simulink library "WBCLibrary"  (R2014b)
settings: Solver=ode45  StartTime=0.0  StopTime=10.0  RelTol=1e-3
undefined symbols (not defined in the file or in its folder): LinkName, localName, ROBOT_DOF, robotName, Ts
undefined symbols (not defined in the file): Tt
libraries: WBCLibrary x10, simulink x1
(part 2 of 2)

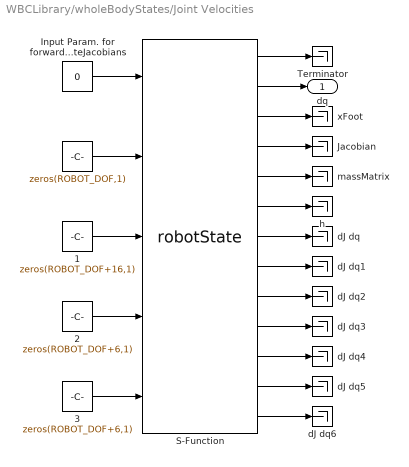
== system WBCLibrary/wholeBodyStates/Joint Velocities ==
  " " : Constant  Value=zeros(ROBOT_DOF,1)  OutDataTypeStr=double  SampleTime=Ts
  " 1" : Constant  Value=zeros(ROBOT_DOF+16,1)  OutDataTypeStr=double  SampleTime=Ts
  " 2" : Constant  Value=zeros(ROBOT_DOF+6,1)  OutDataTypeStr=double  SampleTime=Ts
  " 3" : Constant  Value=zeros(ROBOT_DOF+6,1)  OutDataTypeStr=double  SampleTime=Ts
  "Input Param. for forwardKinematics and computeJacobians " : Constant  Value=0  OutDataTypeStr=int8  SampleTime=Ts
  Jacobian : Terminator
  S-Function : S-Function  FunctionName=robotState  Parameters=val,robotname,localname,linkname  EnableBusSupport=off  mask{val=1, robotname=robotName, localname=localName, linkname='na'}
      mask prompts: val "Value"; robotname "Robot Name (icub - icubSim)"; localname "Module Name"; linkname "Link Name"
  Terminator : Terminator
  dJ dq{,1..6} (7 alike) : Terminator
  h : Terminator
  massMatrix : Terminator
  xFoot : Terminator
  dq : Outport
  wires:
  " "/1 -> S-Function/2
  S-Function/2 -> dq/1
  S-Function/1 -> Terminator/1
  S-Function/3 -> xFoot/1
  "Input Param. for forwardKinematics and computeJacobians "/1 -> S-Function/1
  S-Function/4 -> Jacobian/1
  S-Function/5 -> massMatrix/1
  S-Function/6 -> h/1
  S-Function/7 -> dJ dq/1
  S-Function/8 -> dJ dq1/1
  S-Function/9 -> dJ dq2/1
  S-Function/10 -> dJ dq3/1
  " 1"/1 -> S-Function/3
  " 2"/1 -> S-Function/4
  " 3"/1 -> S-Function/5
  S-Function/11 -> dJ dq4/1
  S-Function/12 -> dJ dq5/1
  S-Function/13 -> dJ dq6/1

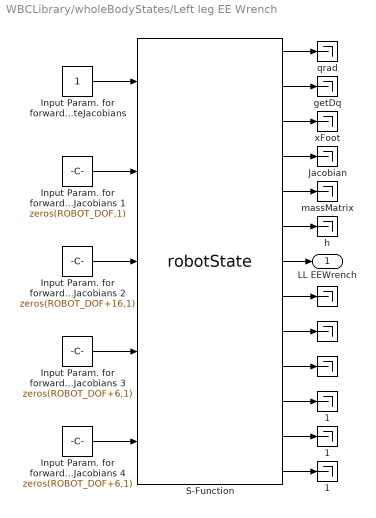
== system WBCLibrary/wholeBodyStates/Left leg EE Wrench ==
  " " : Terminator
  "  " : Terminator
  "   " : Terminator
  "   1" : Terminator
  "  1" : Terminator
  " 1" : Terminator
  "Input Param. for forwardKinematics and computeJacobians " : Constant  OutDataTypeStr=int8  SampleTime=Ts
  Input Param. for forwardKinematics and computeJacobians 1 : Constant  Value=zeros(ROBOT_DOF,1)  OutDataTypeStr=double  SampleTime=Ts
  Input Param. for forwardKinematics and computeJacobians 2 : Constant  Value=zeros(ROBOT_DOF+16,1)  OutDataTypeStr=double  SampleTime=Ts
  Input Param. for forwardKinematics and computeJacobians 3 : Constant  Value=zeros(ROBOT_DOF+6,1)  OutDataTypeStr=double  SampleTime=Ts
  Input Param. for forwardKinematics and computeJacobians 4 : Constant  Value=zeros(ROBOT_DOF+6,1)  OutDataTypeStr=double  SampleTime=Ts
  Jacobian : Terminator
  S-Function : S-Function  FunctionName=robotState  Parameters=val,robotname,localname,linkname  EnableBusSupport=off  mask{val=15, robotname=robotName, localname=localName, linkname='l_sole'}
      mask prompts: val "Value"; robotname "Robot Name (icub - icubSim)"; localname "Module Name"; linkname "Link Name"
  getDq : Terminator
  h : Terminator
  massMatrix : Terminator
  qrad : Terminator
  xFoot : Terminator
  LL EEWrench : Outport
  wires:
  Input Param. for forwardKinematics and computeJacobians 4/1 -> S-Function/5
  Input Param. for forwardKinematics and computeJacobians 3/1 -> S-Function/4
  Input Param. for forwardKinematics and computeJacobians 2/1 -> S-Function/3
  S-Function/10 -> "   "/1
  S-Function/9 -> "  "/1
  S-Function/8 -> " "/1
  S-Function/7 -> LL EEWrench/1
  S-Function/6 -> h/1
  S-Function/5 -> massMatrix/1
  S-Function/4 -> Jacobian/1
  "Input Param. for forwardKinematics and computeJacobians "/1 -> S-Function/1
  S-Function/3 -> xFoot/1
  S-Function/1 -> qrad/1
  S-Function/2 -> getDq/1
  Input Param. for forwardKinematics and computeJacobians 1/1 -> S-Function/2
  S-Function/11 -> " 1"/1
  S-Function/12 -> "  1"/1
  S-Function/13 -> "   1"/1

== system WBCLibrary/wholeBodyStates/Right leg EE Wrench ==
  " " : Constant  Value=zeros(ROBOT_DOF,1)  OutDataTypeStr=double  SampleTime=-1
  " 1" : Constant  Value=zeros(ROBOT_DOF+16,1)  OutDataTypeStr=double  SampleTime=-1
  " 2" : Constant  Value=zeros(ROBOT_DOF+6,1)  OutDataTypeStr=double  SampleTime=-1
  " 3" : Constant  Value=zeros(ROBOT_DOF+6,1)  OutDataTypeStr=double  SampleTime=-1
  "Input Param. for forwardKinematics and computeJacobians " : Constant  Value=0  OutDataTypeStr=int8
  Jacobian : Terminator
  S-Function : S-Function  FunctionName=robotState  Parameters=val,robotname,localname,linkname  EnableBusSupport=off  mask{val=15, robotname=robotName, localname=localName, linkname='r_sole'}
      mask prompts: val "Value"; robotname "Robot Name (icub - icubSim)"; localname "Module Name"; linkname "Link Name"
  Terminator : Terminator
  Terminator1 : Terminator
  dJ dq{1..6} (6 alike) : Terminator
  h : Terminator
  massMatrix : Terminator
  xFoot : Terminator
  RL EEWrench : Outport
  wires:
  " 3"/1 -> S-Function/5
  " 2"/1 -> S-Function/4
  " 1"/1 -> S-Function/3
  S-Function/10 -> dJ dq3/1
  S-Function/9 -> dJ dq2/1
  S-Function/8 -> dJ dq1/1
  S-Function/7 -> RL EEWrench/1
  S-Function/6 -> h/1
  S-Function/5 -> massMatrix/1
  S-Function/4 -> Jacobian/1
  "Input Param. for forwardKinematics and computeJacobians "/1 -> S-Function/1
  S-Function/3 -> xFoot/1
  S-Function/1 -> Terminator/1
  S-Function/2 -> Terminator1/1
  " "/1 -> S-Function/2
  S-Function/13 -> dJ dq6/1
  S-Function/12 -> dJ dq5/1
  S-Function/11 -> dJ dq4/1

== system WBCLibrary/wholeBodyStates/dq_b + dq_j ==
  Joint Velocities : WBCLibrary/wholeBodyStates/Joint Velocities  robotName=robotName  localName=localName
  Left Foot Jacobian : WBCLibrary/wholeBodyModel/Jacobians/Left Foot Jacobian  robotName=robotName  localName=localName
  Mux : Mux  Inputs=2
  Right Foot Jacobian : WBCLibrary/wholeBodyModel/Jacobians/Right Foot Jacobian  robotName=robotName  localName=localName
  baseVelocity : WBCLibrary/Utilities/baseVelocity
  dq : Outport
  wires:
  Mux/1 -> dq/1
  Joint Velocities/1 -> Mux/2, baseVelocity/3
  baseVelocity/1 -> Mux/1
  Right Foot Jacobian/1 -> baseVelocity/1
  Left Foot Jacobian/1 -> baseVelocity/2

== system WBCLibrary/wholeBodyStates/q_b + q_j ==
  Constant1 : Constant  Value=zeros(16,1)
  Joint Angles : WBCLibrary/wholeBodyStates/Joint Angles  robotName=robotName  localName=localName
  Mux : Mux  Inputs=2
  q : Outport
  wires:
  Constant1/1 -> Mux/1
  Joint Angles/1 -> Mux/2
  Mux/1 -> q/1

== system WBCLibrary/wholeBodyModel/Dynamics/Cent Momentum ==
  q : Inport
  dq : Inport  Port=2
  RightFoot : Constant  Value=0  OutDataTypeStr=int8  SampleTime=Ts
  S-Function : S-Function  FunctionName=robotState  Parameters=14,robotName,localName,'na'  EnableBusSupport=off
  Terminator{,1..11} (12 alike) : Terminator
  dummy : Constant  Value=zeros(ROBOT_DOF,1)  OutDataTypeStr=double  SampleTime=Ts
  dummy3 : Constant  Value=zeros(ROBOT_DOF+6,1)  OutDataTypeStr=double  SampleTime=Ts
  H : Outport
  wires:
  S-Function/13 -> H/1
  dummy3/1 -> S-Function/5
  dq/1 -> S-Function/4
  q/1 -> S-Function/3
  dummy/1 -> S-Function/2
  RightFoot/1 -> S-Function/1
  S-Function/12 -> Terminator11/1
  S-Function/11 -> Terminator10/1
  S-Function/10 -> Terminator9/1
  S-Function/9 -> Terminator8/1
  S-Function/8 -> Terminator7/1
  S-Function/7 -> Terminator6/1
  S-Function/6 -> Terminator5/1
  S-Function/5 -> Terminator4/1
  S-Function/4 -> Terminator3/1
  S-Function/3 -> Terminator2/1
  S-Function/2 -> Terminator1/1
  S-Function/1 -> Terminator/1

== system WBCLibrary/wholeBodyModel/Dynamics/Inverse Dynamics ==
  q : Inport
  dq : Inport  Port=2
  ddq : Inport  Port=3
  Constant : Constant  Value=zeros(ROBOT_DOF,1)  OutDataTypeStr=double  SampleTime=Ts
  Constant2 : Constant  Value=0  OutDataTypeStr=int8  SampleTime=Ts
  S-Function : S-Function  FunctionName=robotState  Parameters=12,robotName,localName,'na'  EnableBusSupport=off
  Terminator{,1..11} (12 alike) : Terminator
  genTau : Outport
  wires:
  S-Function/10 -> genTau/1
  S-Function/9 -> Terminator8/1
  Constant/1 -> S-Function/2
  Constant2/1 -> S-Function/1
  q/1 -> S-Function/3
  dq/1 -> S-Function/4
  ddq/1 -> S-Function/5
  S-Function/1 -> Terminator/1
  S-Function/2 -> Terminator1/1
  S-Function/3 -> Terminator2/1
  S-Function/4 -> Terminator3/1
  S-Function/5 -> Terminator4/1
  S-Function/6 -> Terminator5/1
  S-Function/7 -> Terminator6/1
  S-Function/8 -> Terminator7/1
  S-Function/11 -> Terminator9/1
  S-Function/12 -> Terminator10/1
  S-Function/13 -> Terminator11/1

== system WBCLibrary/wholeBodyModel/Dynamics/computeh ==
  q : Inport
  dq : Inport  Port=2
  " " : Terminator
  "  " : Terminator
  "  1" : Terminator
  "  2" : Terminator
  Constant : Constant  Value=0  OutDataTypeStr=int8  SampleTime=Ts
  Constant1 : Constant  Value=zeros(ROBOT_DOF,1)  OutDataTypeStr=double  SampleTime=Ts
  Constant4 : Constant  Value=zeros(ROBOT_DOF+6,1)  OutDataTypeStr=double  SampleTime=Ts
  S-Function : S-Function  FunctionName=robotState  Parameters=val,robotname,localname,'na'  EnableBusSupport=off
  h{1..8} (8 alike) : Terminator
  h : Outport
  wires:
  Constant/1 -> S-Function/1
  Constant1/1 -> S-Function/2
  S-Function/1 -> h1/1
  S-Function/2 -> h2/1
  S-Function/3 -> h3/1
  S-Function/4 -> h4/1
  S-Function/5 -> "  "/1
  S-Function/7 -> " "/1
  S-Function/6 -> h/1
  S-Function/8 -> h5/1
  S-Function/9 -> h6/1
  S-Function/10 -> "  1"/1
  q/1 -> S-Function/3
  dq/1 -> S-Function/4
  Constant4/1 -> S-Function/5
  S-Function/11 -> h7/1
  S-Function/12 -> h8/1
  S-Function/13 -> "  2"/1

== system WBCLibrary/wholeBodyModel/Dynamics/dJ*dq LeftArm ==
  q : Inport
  dq : Inport  Port=2
  LeftFoot : Constant  Value=4  OutDataTypeStr=int8  SampleTime=Ts
  S-Function : S-Function  FunctionName=robotState  Parameters=val,robotName,localName,'na'  EnableBusSupport=off
  Terminator{,1..11} (12 alike) : Terminator
  dummy : Constant  Value=zeros(ROBOT_DOF,1)  OutDataTypeStr=double  SampleTime=Ts
  dummy3 : Constant  Value=zeros(ROBOT_DOF+6,1)  OutDataTypeStr=double  SampleTime=Ts
  dJdqLA : Outport
  wires:
  dummy3/1 -> S-Function/5
  dq/1 -> S-Function/4
  q/1 -> S-Function/3
  S-Function/10 -> Terminator8/1
  S-Function/9 -> Terminator7/1
  S-Function/8 -> Terminator6/1
  LeftFoot/1 -> S-Function/1
  dummy/1 -> S-Function/2
  S-Function/7 -> dJdqLA/1
  S-Function/1 -> Terminator/1
  S-Function/2 -> Terminator1/1
  S-Function/3 -> Terminator2/1
  S-Function/4 -> Terminator3/1
  S-Function/5 -> Terminator4/1
  S-Function/6 -> Terminator5/1
  S-Function/11 -> Terminator9/1
  S-Function/12 -> Terminator10/1
  S-Function/13 -> Terminator11/1

== system WBCLibrary/wholeBodyModel/Dynamics/dJ*dq LeftFoot ==
  q : Inport
  dq : Inport  Port=2
  LeftFoot : Constant  OutDataTypeStr=int8  SampleTime=Ts
  S-Function : S-Function  FunctionName=robotState  Parameters=val,robotName,localName,'na'  EnableBusSupport=off
  Terminator{,1..11} (12 alike) : Terminator
  dummy : Constant  Value=zeros(ROBOT_DOF,1)  OutDataTypeStr=double  SampleTime=Ts
  dummy3 : Constant  Value=zeros(ROBOT_DOF+6,1)  OutDataTypeStr=double  SampleTime=Ts
  dJdqLF : Outport
  wires:
  S-Function/6 -> Terminator5/1
  S-Function/5 -> Terminator4/1
  S-Function/4 -> Terminator3/1
  S-Function/3 -> Terminator2/1
  S-Function/2 -> Terminator1/1
  S-Function/1 -> Terminator/1
  S-Function/7 -> dJdqLF/1
  dummy/1 -> S-Function/2
  LeftFoot/1 -> S-Function/1
  S-Function/8 -> Terminator6/1
  S-Function/9 -> Terminator7/1
  S-Function/10 -> Terminator8/1
  q/1 -> S-Function/3
  dq/1 -> S-Function/4
  dummy3/1 -> S-Function/5
  S-Function/11 -> Terminator9/1
  S-Function/12 -> Terminator10/1
  S-Function/13 -> Terminator11/1

== system WBCLibrary/wholeBodyModel/Dynamics/dJ*dq Link ==
  q : Inport
  dq : Inport  Port=2
  RightFoot : Constant  Value=0  OutDataTypeStr=int8  SampleTime=Ts
  S-Function : S-Function  FunctionName=robotState  Parameters=val,robotName,localName,LinkName  EnableBusSupport=off
  Terminator{,1..11} (12 alike) : Terminator
  dummy : Constant  Value=zeros(ROBOT_DOF,1)  OutDataTypeStr=double  SampleTime=Ts
  dummy3 : Constant  Value=zeros(ROBOT_DOF+6,1)  OutDataTypeStr=double  SampleTime=Ts
  dJdq : Outport
  wires:
  S-Function/13 -> Terminator11/1
  S-Function/12 -> Terminator10/1
  S-Function/11 -> Terminator9/1
  dummy3/1 -> S-Function/5
  dq/1 -> S-Function/4
  q/1 -> S-Function/3
  S-Function/10 -> Terminator8/1
  S-Function/9 -> Terminator7/1
  S-Function/8 -> Terminator6/1
  RightFoot/1 -> S-Function/1
  dummy/1 -> S-Function/2
  S-Function/7 -> dJdq/1
  S-Function/1 -> Terminator/1
  S-Function/2 -> Terminator1/1
  S-Function/3 -> Terminator2/1
  S-Function/4 -> Terminator3/1
  S-Function/5 -> Terminator4/1
  S-Function/6 -> Terminator5/1

== system WBCLibrary/wholeBodyModel/Dynamics/dJ*dq RightArm ==
  q : Inport
  dq : Inport  Port=2
  RightFoot : Constant  Value=3  OutDataTypeStr=int8  SampleTime=Ts
  S-Function : S-Function  FunctionName=robotState  Parameters=val,robotName,localName,'na'  EnableBusSupport=off
  Terminator{,1..11} (12 alike) : Terminator
  dummy : Constant  Value=zeros(ROBOT_DOF,1)  OutDataTypeStr=double  SampleTime=Ts
  dummy3 : Constant  Value=zeros(ROBOT_DOF+6,1)  OutDataTypeStr=double  SampleTime=Ts
  dJdqRA : Outport
  wires:
  dummy3/1 -> S-Function/5
  dq/1 -> S-Function/4
  q/1 -> S-Function/3
  S-Function/10 -> Terminator8/1
  S-Function/9 -> Terminator7/1
  S-Function/8 -> Terminator6/1
  RightFoot/1 -> S-Function/1
  dummy/1 -> S-Function/2
  S-Function/7 -> dJdqRA/1
  S-Function/1 -> Terminator/1
  S-Function/2 -> Terminator1/1
  S-Function/3 -> Terminator2/1
  S-Function/4 -> Terminator3/1
  S-Function/5 -> Terminator4/1
  S-Function/6 -> Terminator5/1
  S-Function/11 -> Terminator9/1
  S-Function/12 -> Terminator10/1
  S-Function/13 -> Terminator11/1

== system WBCLibrary/wholeBodyModel/Dynamics/dJ*dq RightFoot ==
  q : Inport
  dq : Inport  Port=2
  RightFoot : Constant  Value=0  OutDataTypeStr=int8  SampleTime=Ts
  S-Function : S-Function  FunctionName=robotState  Parameters=val,robotName,localName,'na'  EnableBusSupport=off
  Terminator{,1..11} (12 alike) : Terminator
  dummy : Constant  Value=zeros(ROBOT_DOF,1)  OutDataTypeStr=double  SampleTime=Ts
  dummy3 : Constant  Value=zeros(ROBOT_DOF+6,1)  OutDataTypeStr=double  SampleTime=Ts
  dJdqRF : Outport
  wires:
  S-Function/6 -> Terminator5/1
  S-Function/5 -> Terminator4/1
  S-Function/4 -> Terminator3/1
  S-Function/3 -> Terminator2/1
  S-Function/2 -> Terminator1/1
  S-Function/1 -> Terminator/1
  S-Function/7 -> dJdqRF/1
  dummy/1 -> S-Function/2
  RightFoot/1 -> S-Function/1
  S-Function/8 -> Terminator6/1
  S-Function/9 -> Terminator7/1
  S-Function/10 -> Terminator8/1
  q/1 -> S-Function/3
  dq/1 -> S-Function/4
  dummy3/1 -> S-Function/5
  S-Function/11 -> Terminator9/1
  S-Function/12 -> Terminator10/1
  S-Function/13 -> Terminator11/1

== system WBCLibrary/wholeBodyModel/Dynamics/massMatrix ==
  q : Inport
  Reshape : Reshape  OutputDimensionality=Customize  OutputDimensions=[ROBOT_DOF+6,ROBOT_DOF+6]
  massMatrix : Subsystem
  M : Outport
  wires:
  Reshape/1 -> M/1
  massMatrix/1(massMatrix) -> Reshape/1
  q/1 -> massMatrix/1(q)

== system WBCLibrary/wholeBodyModel/Forward Kinematics/COMFwdKin  ==
  "Input Param. for forwardKinematics and computeJacobians " : Constant  Value=2  OutDataTypeStr=int8  SampleTime=Ts
  Input Param. for forwardKinematics and computeJacobians 1 : Constant  Value=zeros(ROBOT_DOF,1)  OutDataTypeStr=double  SampleTime=Ts
  Input Param. for forwardKinematics and computeJacobians 2 : Constant  Value=zeros(ROBOT_DOF+16,1)  OutDataTypeStr=double  SampleTime=Ts
  Input Param. for forwardKinematics and computeJacobians 3 : Constant  Value=zeros(ROBOT_DOF+6,1)  OutDataTypeStr=double  SampleTime=Ts
  Input Param. for forwardKinematics and computeJacobians 4 : Constant  Value=zeros(ROBOT_DOF+6,1)  OutDataTypeStr=double  SampleTime=Ts
  Jacobian : Terminator
  S-Function : S-Function  FunctionName=robotState  Parameters=val,robotname,localname,linkname  EnableBusSupport=off  mask{val=2, robotname=robotName, localname=localName, linkname='na'}
      mask prompts: val "Value"; robotname "Robot Name (icub - icubSim)"; localname "Module Name"; linkname "Link Name"
  dJ dq{,1..6} (7 alike) : Terminator
  getDq : Terminator
  h : Terminator
  massMatrix : Terminator
  qrad : Terminator
  xCOM : Outport
  wires:
  S-Function/4 -> Jacobian/1
  "Input Param. for forwardKinematics and computeJacobians "/1 -> S-Function/1
  S-Function/3 -> xCOM/1
  S-Function/1 -> qrad/1
  S-Function/2 -> getDq/1
  Input Param. for forwardKinematics and computeJacobians 1/1 -> S-Function/2
  S-Function/5 -> massMatrix/1
  S-Function/6 -> h/1
  S-Function/7 -> dJ dq/1
  S-Function/8 -> dJ dq1/1
  S-Function/9 -> dJ dq2/1
  S-Function/10 -> dJ dq3/1
  Input Param. for forwardKinematics and computeJacobians 2/1 -> S-Function/3
  Input Param. for forwardKinematics and computeJacobians 3/1 -> S-Function/4
  Input Param. for forwardKinematics and computeJacobians 4/1 -> S-Function/5
  S-Function/11 -> dJ dq4/1
  S-Function/12 -> dJ dq5/1
  S-Function/13 -> dJ dq6/1

== system WBCLibrary/wholeBodyModel/Forward Kinematics/LeftFootFwdKin ==
  "Input Param. for forwardKinematics and computeJacobians " : Constant  OutDataTypeStr=int8  SampleTime=Ts
  Input Param. for forwardKinematics and computeJacobians 1 : Constant  Value=zeros(ROBOT_DOF,1)  OutDataTypeStr=double  SampleTime=Ts
  Input Param. for forwardKinematics and computeJacobians 2 : Constant  Value=zeros(ROBOT_DOF+16,1)  OutDataTypeStr=double  SampleTime=Ts
  Input Param. for forwardKinematics and computeJacobians 3 : Constant  Value=zeros(ROBOT_DOF+6,1)  OutDataTypeStr=double  SampleTime=Ts
  Input Param. for forwardKinematics and computeJacobians 4 : Constant  Value=zeros(ROBOT_DOF+6,1)  OutDataTypeStr=double  SampleTime=Ts
  Jacobian : Terminator
  S-Function : S-Function  FunctionName=robotState  Parameters=val,robotname,localname,linkname  EnableBusSupport=off  mask{val=2, robotname=robotName, localname=localName, linkname='na'}
      mask prompts: val "Value"; robotname "Robot Name (icub - icubSim)"; localname "Module Name"; linkname "Link Name"
  dJ dq{,1..6} (7 alike) : Terminator
  getDq : Terminator
  h : Terminator
  massMatrix : Terminator
  qrad : Terminator
  xLeftFoot : Outport
  wires:
  S-Function/4 -> Jacobian/1
  "Input Param. for forwardKinematics and computeJacobians "/1 -> S-Function/1
  S-Function/3 -> xLeftFoot/1
  S-Function/1 -> qrad/1
  S-Function/2 -> getDq/1
  Input Param. for forwardKinematics and computeJacobians 1/1 -> S-Function/2
  S-Function/5 -> massMatrix/1
  S-Function/6 -> h/1
  S-Function/7 -> dJ dq/1
  Input Param. for forwardKinematics and computeJacobians 2/1 -> S-Function/3
  Input Param. for forwardKinematics and computeJacobians 3/1 -> S-Function/4
  Input Param. for forwardKinematics and computeJacobians 4/1 -> S-Function/5
  S-Function/8 -> dJ dq1/1
  S-Function/9 -> dJ dq2/1
  S-Function/10 -> dJ dq3/1
  S-Function/11 -> dJ dq4/1
  S-Function/12 -> dJ dq5/1
  S-Function/13 -> dJ dq6/1

== system WBCLibrary/wholeBodyModel/Forward Kinematics/LeftHandFwdKin ==
  "Input Param. for forwardKinematics and computeJacobians " : Constant  Value=4  OutDataTypeStr=int8  SampleTime=Ts
  Input Param. for forwardKinematics and computeJacobians 1 : Constant  Value=zeros(ROBOT_DOF,1)  OutDataTypeStr=double  SampleTime=Ts
  Input Param. for forwardKinematics and computeJacobians 2 : Constant  Value=zeros(ROBOT_DOF+16,1)  OutDataTypeStr=double  SampleTime=Ts
  Input Param. for forwardKinematics and computeJacobians 3 : Constant  Value=zeros(ROBOT_DOF+6,1)  OutDataTypeStr=double  SampleTime=Ts
  Input Param. for forwardKinematics and computeJacobians 4 : Constant  Value=zeros(ROBOT_DOF+6,1)  OutDataTypeStr=double  SampleTime=Ts
  Jacobian : Terminator
  S-Function : S-Function  FunctionName=robotState  Parameters=val,robotname,localname,linkname  EnableBusSupport=off  mask{val=2, robotname=robotName, localname=localName, linkname='na'}
      mask prompts: val "Value"; robotname "Robot Name (icub - icubSim)"; localname "Module Name"; linkname "Link Name"
  dJ dq{,1..6} (7 alike) : Terminator
  getDq : Terminator
  h : Terminator
  massMatrix : Terminator
  qrad : Terminator
  xLeftHand : Outport
  wires:
  Input Param. for forwardKinematics and computeJacobians 4/1 -> S-Function/5
  Input Param. for forwardKinematics and computeJacobians 3/1 -> S-Function/4
  Input Param. for forwardKinematics and computeJacobians 2/1 -> S-Function/3
  S-Function/10 -> dJ dq3/1
  S-Function/9 -> dJ dq2/1
  S-Function/8 -> dJ dq1/1
  S-Function/4 -> Jacobian/1
  "Input Param. for forwardKinematics and computeJacobians "/1 -> S-Function/1
  S-Function/3 -> xLeftHand/1
  S-Function/1 -> qrad/1
  S-Function/2 -> getDq/1
  Input Param. for forwardKinematics and computeJacobians 1/1 -> S-Function/2
  S-Function/5 -> massMatrix/1
  S-Function/6 -> h/1
  S-Function/7 -> dJ dq/1
  S-Function/11 -> dJ dq4/1
  S-Function/12 -> dJ dq5/1
  S-Function/13 -> dJ dq6/1

== system WBCLibrary/wholeBodyModel/Forward Kinematics/LinkFwdKin ==
  "Input Param. for forwardKinematics and computeJacobians " : Constant  Value=2  OutDataTypeStr=int8  SampleTime=Ts
  Input Param. for forwardKinematics and computeJacobians 1 : Constant  Value=zeros(ROBOT_DOF,1)  OutDataTypeStr=double  SampleTime=Ts
  Input Param. for forwardKinematics and computeJacobians 2 : Constant  Value=zeros(ROBOT_DOF+16,1)  OutDataTypeStr=double  SampleTime=Ts
  Input Param. for forwardKinematics and computeJacobians 3 : Constant  Value=zeros(ROBOT_DOF+6,1)  OutDataTypeStr=double  SampleTime=Ts
  Input Param. for forwardKinematics and computeJacobians 4 : Constant  Value=zeros(ROBOT_DOF+6,1)  OutDataTypeStr=double  SampleTime=Ts
  Jacobian : Terminator
  S-Function : S-Function  FunctionName=robotState  Parameters=17,robotname,localname,LinkName  EnableBusSupport=off
  dJ dq{,1..6} (7 alike) : Terminator
  getDq : Terminator
  h : Terminator
  massMatrix : Terminator
  qrad : Terminator
  x : Outport
  wires:
  Input Param. for forwardKinematics and computeJacobians 4/1 -> S-Function/5
  Input Param. for forwardKinematics and computeJacobians 3/1 -> S-Function/4
  Input Param. for forwardKinematics and computeJacobians 2/1 -> S-Function/3
  S-Function/10 -> dJ dq3/1
  S-Function/9 -> dJ dq2/1
  S-Function/8 -> dJ dq1/1
  S-Function/7 -> dJ dq/1
  S-Function/6 -> h/1
  S-Function/5 -> massMatrix/1
  Input Param. for forwardKinematics and computeJacobians 1/1 -> S-Function/2
  S-Function/2 -> getDq/1
  S-Function/1 -> qrad/1
  S-Function/3 -> x/1
  "Input Param. for forwardKinematics and computeJacobians "/1 -> S-Function/1
  S-Function/4 -> Jacobian/1
  S-Function/11 -> dJ dq4/1
  S-Function/12 -> dJ dq5/1
  S-Function/13 -> dJ dq6/1

== system WBCLibrary/wholeBodyModel/Forward Kinematics/RightFootFwdKin ==
  "Input Param. for forwardKinematics and computeJacobians " : Constant  Value=0  OutDataTypeStr=int8  SampleTime=Ts
  Input Param. for forwardKinematics and computeJacobians 1 : Constant  Value=zeros(ROBOT_DOF,1)  OutDataTypeStr=double  SampleTime=Ts
  Input Param. for forwardKinematics and computeJacobians 2 : Constant  Value=zeros(ROBOT_DOF+16,1)  OutDataTypeStr=double  SampleTime=Ts
  Input Param. for forwardKinematics and computeJacobians 3 : Constant  Value=zeros(ROBOT_DOF+6,1)  OutDataTypeStr=double  SampleTime=Ts
  Input Param. for forwardKinematics and computeJacobians 4 : Constant  Value=zeros(ROBOT_DOF+6,1)  OutDataTypeStr=double  SampleTime=Ts
  Jacobian : Terminator
  S-Function : S-Function  FunctionName=robotState  Parameters=val,robotname,localname,linkname  EnableBusSupport=off  mask{val=2, robotname=robotName, localname=localName, linkname='na'}
      mask prompts: val "Value"; robotname "Robot Name (icub - icubSim)"; localname "Module Name"; linkname "Link Name"
  dJ dq{,1..6} (7 alike) : Terminator
  getDq : Terminator
  h : Terminator
  massMatrix : Terminator
  qrad : Terminator
  xRightFoot : Outport
  wires:
  S-Function/7 -> dJ dq/1
  S-Function/6 -> h/1
  S-Function/5 -> massMatrix/1
  Input Param. for forwardKinematics and computeJacobians 1/1 -> S-Function/2
  S-Function/2 -> getDq/1
  S-Function/1 -> qrad/1
  S-Function/3 -> xRightFoot/1
  "Input Param. for forwardKinematics and computeJacobians "/1 -> S-Function/1
  S-Function/4 -> Jacobian/1
  S-Function/8 -> dJ dq1/1
  S-Function/9 -> dJ dq2/1
  S-Function/10 -> dJ dq3/1
  Input Param. for forwardKinematics and computeJacobians 2/1 -> S-Function/3
  Input Param. for forwardKinematics and computeJacobians 3/1 -> S-Function/4
  Input Param. for forwardKinematics and computeJacobians 4/1 -> S-Function/5
  S-Function/11 -> dJ dq4/1
  S-Function/12 -> dJ dq5/1
  S-Function/13 -> dJ dq6/1

== system WBCLibrary/wholeBodyModel/Forward Kinematics/RightHandFwdKin ==
  "Input Param. for forwardKinematics and computeJacobians " : Constant  Value=3  OutDataTypeStr=int8  SampleTime=Ts
  Input Param. for forwardKinematics and computeJacobians 1 : Constant  Value=zeros(ROBOT_DOF,1)  OutDataTypeStr=double  SampleTime=Ts
  Input Param. for forwardKinematics and computeJacobians 2 : Constant  Value=zeros(ROBOT_DOF+16,1)  OutDataTypeStr=double  SampleTime=Ts
  Input Param. for forwardKinematics and computeJacobians 3 : Constant  Value=zeros(ROBOT_DOF+6,1)  OutDataTypeStr=double  SampleTime=Ts
  Input Param. for forwardKinematics and computeJacobians 4 : Constant  Value=zeros(ROBOT_DOF+6,1)  OutDataTypeStr=double  SampleTime=Ts
  Jacobian : Terminator
  S-Function : S-Function  FunctionName=robotState  Parameters=val,robotname,localname,linkname  EnableBusSupport=off  mask{val=2, robotname=robotName, localname=localName, linkname='na'}
      mask prompts: val "Value"; robotname "Robot Name (icub - icubSim)"; localname "Module Name"; linkname "Link Name"
  dJ dq{,1..6} (7 alike) : Terminator
  getDq : Terminator
  h : Terminator
  massMatrix : Terminator
  qrad : Terminator
  xRightHand : Outport
  wires:
  S-Function/7 -> dJ dq/1
  S-Function/6 -> h/1
  S-Function/5 -> massMatrix/1
  Input Param. for forwardKinematics and computeJacobians 1/1 -> S-Function/2
  S-Function/2 -> getDq/1
  S-Function/1 -> qrad/1
  S-Function/3 -> xRightHand/1
  "Input Param. for forwardKinematics and computeJacobians "/1 -> S-Function/1
  S-Function/4 -> Jacobian/1
  S-Function/8 -> dJ dq1/1
  S-Function/9 -> dJ dq2/1
  S-Function/10 -> dJ dq3/1
  Input Param. for forwardKinematics and computeJacobians 2/1 -> S-Function/3
  Input Param. for forwardKinematics and computeJacobians 3/1 -> S-Function/4
  Input Param. for forwardKinematics and computeJacobians 4/1 -> S-Function/5
  S-Function/12 -> dJ dq5/1
  S-Function/13 -> dJ dq6/1
  S-Function/11 -> dJ dq4/1

== system WBCLibrary/wholeBodyModel/Jacobians/Center of Mass Jacobian ==
  COM Jacobian : Subsystem
  rs1 : Reshape  OutputDimensionality=Customize  OutputDimensions=[6, ROBOT_DOF+6]
  COMJacob : Outport
  wires:
  rs1/1 -> COMJacob/1
  COM Jacobian/1(Jacobian) -> rs1/1

== system WBCLibrary/wholeBodyModel/Jacobians/Left Foot Jacobian ==
  Left Foot Jacobian : Subsystem
  rs2 : Reshape  OutputDimensionality=Customize  OutputDimensions=[6,ROBOT_DOF+6]
  LFootJacob : Outport
  wires:
  Left Foot Jacobian/1(Jacobian) -> rs2/1
  rs2/1 -> LFootJacob/1

== system WBCLibrary/wholeBodyModel/Jacobians/Left Hand Jacobian ==
  Left Hand Jacobian : Subsystem
  rs2 : Reshape  OutputDimensionality=Customize  OutputDimensions=[6, ROBOT_DOF+6]
  LHandJacob : Outport
  wires:
  rs2/1 -> LHandJacob/1
  Left Hand Jacobian/1(Jacobian) -> rs2/1

== system WBCLibrary/wholeBodyModel/Jacobians/Link Jacobian ==
  Link Jacobian : Subsystem
  rs2 : Reshape  OutputDimensionality=Customize  OutputDimensions=[6, ROBOT_DOF+6]
  Jacobian : Outport
  wires:
  rs2/1 -> Jacobian/1
  Link Jacobian/1(Jacobian) -> rs2/1

== system WBCLibrary/wholeBodyModel/Jacobians/Right Foot Jacobian ==
  Right Foot Jacobian : Subsystem
  rs1 : Reshape  OutputDimensionality=Customize  OutputDimensions=[6, ROBOT_DOF+6]
  RFootJacob : Outport
  wires:
  Right Foot Jacobian/1(Jacobian) -> rs1/1
  rs1/1 -> RFootJacob/1

== system WBCLibrary/wholeBodyModel/Jacobians/Right Hand Jacobian ==
  Right Hand Jacobian : Subsystem
  rs1 : Reshape  OutputDimensionality=Customize  OutputDimensions=[6, ROBOT_DOF+6]
  RHandJacob : Outport
  wires:
  rs1/1 -> RHandJacob/1
  Right Hand Jacobian/1(Jacobian) -> rs1/1

== system WBCLibrary/wholeBodyStates/DUMMY Joint Torques/tau from ports ==
  Mux : Mux  Inputs=5
  Mux1 : Mux  Inputs=5
  Mux2 : Mux  Inputs=3
  Mux4 : Mux  Inputs=6
  Mux5 : Mux  Inputs=6
  yarp armL : WBCLibrary/Utilities/yarp read  from=['/' robotName '/left_arm/analog:o/torques']  to='...'  num=5  blocking=off  timestamp=off
  yarp armR : WBCLibrary/Utilities/yarp read  from=['/' robotName '/right_arm/analog:o/torques']  to='...'  num=5  blocking=off  timestamp=off
  yarp legL : WBCLibrary/Utilities/yarp read  from=['/' robotName '/left_leg/analog:o/torques']  to='...'  num=6  blocking=off  timestamp=off
  yarp legR : WBCLibrary/Utilities/yarp read  from=['/' robotName '/right_leg/analog:o/torques']  to='...'  num=6  blocking=off  timestamp=off
  yarp torso : WBCLibrary/Utilities/yarp read  from=['/' robotName '/torso/analog:o/torques']  to='...'  num=3  blocking=off  timestamp=off
  torso : Outport
  leftArm : Outport  Port=2
  rightArm : Outport  Port=3
  leftLeg : Outport  Port=4
  rightLeg : Outport  Port=5
  wires:
  yarp legR/6 -> Mux4/6
  yarp legR/5 -> Mux4/5
  yarp legR/4 -> Mux4/4
  yarp legR/3 -> Mux4/3
  yarp legR/2 -> Mux4/2
  yarp legR/1 -> Mux4/1
  yarp legL/6 -> Mux5/6
  yarp legL/5 -> Mux5/5
  yarp legL/4 -> Mux5/4
  yarp legL/3 -> Mux5/3
  yarp legL/2 -> Mux5/2
  yarp legL/1 -> Mux5/1
  yarp armR/5 -> Mux/5
  yarp armR/4 -> Mux/4
  yarp armR/3 -> Mux/3
  yarp armR/2 -> Mux/2
  yarp armR/1 -> Mux/1
  yarp armL/5 -> Mux1/5
  yarp armL/4 -> Mux1/4
  yarp armL/3 -> Mux1/3
  yarp armL/2 -> Mux1/2
  yarp armL/1 -> Mux1/1
  yarp torso/1 -> Mux2/1
  yarp torso/2 -> Mux2/2
  yarp torso/3 -> Mux2/3
  Mux2/1 -> torso/1
  Mux1/1 -> leftArm/1
  Mux/1 -> rightArm/1
  Mux5/1 -> leftLeg/1
  Mux4/1 -> rightLeg/1

== system WBCLibrary/wholeBodyStates/DUMMY Joint Torques/yarp to WBI ==
  torso : Inport
  leftArm : Inport  Port=2
  rightArm : Inport  Port=3
  leftLeg : Inport  Port=4
  rightLeg : Inport  Port=5
  Mux3 : Mux  Inputs=5
  Selector : Selector  InputPortWidth=3  Indices=[3 2 1]
  WBI ordered : Outport
  wires:
  Selector/1 -> Mux3/1
  torso/1 -> Selector/1
  leftArm/1 -> Mux3/2
  rightArm/1 -> Mux3/3
  Mux3/1 -> WBI ordered/1
  leftLeg/1 -> Mux3/4
  rightLeg/1 -> Mux3/5

== system WBCLibrary/wholeBodyModel/Dynamics/massMatrix/massMatrix ==
  q : Inport
  Constant : Constant  Value=0  OutDataTypeStr=int8  SampleTime=Ts
  Constant1 : Constant  Value=zeros(ROBOT_DOF,1)  OutDataTypeStr=double  SampleTime=Ts
  Constant3 : Constant  Value=zeros(ROBOT_DOF+6,1)  OutDataTypeStr=double  SampleTime=Ts
  Constant4 : Constant  Value=zeros(ROBOT_DOF+6,1)  OutDataTypeStr=double  SampleTime=Ts
  S-Function : S-Function  FunctionName=robotState  Parameters=val,robotname,localname,'na'  EnableBusSupport=off
  Terminator{,1..11} (12 alike) : Terminator
  massMatrix : Outport
  wires:
  S-Function/7 -> Terminator5/1
  S-Function/6 -> Terminator4/1
  S-Function/4 -> Terminator3/1
  S-Function/3 -> Terminator2/1
  S-Function/2 -> Terminator1/1
  S-Function/1 -> Terminator/1
  S-Function/5 -> massMatrix/1
  Constant1/1 -> S-Function/2
  Constant/1 -> S-Function/1
  S-Function/8 -> Terminator6/1
  S-Function/9 -> Terminator7/1
  S-Function/10 -> Terminator8/1
  q/1 -> S-Function/3
  Constant3/1 -> S-Function/4
  Constant4/1 -> S-Function/5
  S-Function/11 -> Terminator9/1
  S-Function/12 -> Terminator10/1
  S-Function/13 -> Terminator11/1

== system WBCLibrary/wholeBodyModel/Jacobians/Center of Mass Jacobian/COM Jacobian ==
  "Input Param. for forwardKinematics and computeJacobians " : Constant  Value=2  OutDataTypeStr=int8  SampleTime=Ts
  Input Param. for forwardKinematics and computeJacobians 1 : Constant  Value=zeros(ROBOT_DOF,1)  OutDataTypeStr=double  SampleTime=Ts
  Input Param. for forwardKinematics and computeJacobians 2 : Constant  Value=zeros(ROBOT_DOF+16,1)  OutDataTypeStr=double  SampleTime=Ts
  Input Param. for forwardKinematics and computeJacobians 3 : Constant  Value=zeros(ROBOT_DOF+6,1)  OutDataTypeStr=double  SampleTime=Ts
  Input Param. for forwardKinematics and computeJacobians 4 : Constant  Value=zeros(ROBOT_DOF+6,1)  OutDataTypeStr=double  SampleTime=Ts
  S-Function : S-Function  FunctionName=robotState  Parameters=val,robotname,localname,linkname  EnableBusSupport=off  mask{val=3, robotname=robotName, localname=localName, linkname='na'}
      mask prompts: val "Value"; robotname "Robot Name (icub - icubSim)"; localname "Module Name"; linkname "Link Name"
  Terminator{1..6} (6 alike) : Terminator
  dqRad : Terminator
  massMatrix : Terminator
  massMatrix1 : Terminator
  massMatrix2 : Terminator
  qRad : Terminator
  x : Terminator
  Jacobian : Outport
  wires:
  S-Function/7 -> Terminator5/1
  S-Function/6 -> Terminator4/1
  S-Function/5 -> massMatrix/1
  S-Function/2 -> dqRad/1
  S-Function/1 -> qRad/1
  S-Function/3 -> x/1
  "Input Param. for forwardKinematics and computeJacobians "/1 -> S-Function/1
  S-Function/4 -> Jacobian/1
  Input Param. for forwardKinematics and computeJacobians 1/1 -> S-Function/2
  S-Function/8 -> massMatrix1/1
  S-Function/9 -> Terminator1/1
  S-Function/10 -> Terminator2/1
  Input Param. for forwardKinematics and computeJacobians 2/1 -> S-Function/3
  Input Param. for forwardKinematics and computeJacobians 3/1 -> S-Function/4
  Input Param. for forwardKinematics and computeJacobians 4/1 -> S-Function/5
  S-Function/11 -> massMatrix2/1
  S-Function/12 -> Terminator3/1
  S-Function/13 -> Terminator6/1

== system WBCLibrary/wholeBodyModel/Jacobians/Left Foot Jacobian/Left Foot Jacobian ==
  "Input Param. for forwardKinematics and computeJacobians " : Constant  OutDataTypeStr=int8  SampleTime=Ts
  Input Param. for forwardKinematics and computeJacobians 1 : Constant  Value=zeros(ROBOT_DOF,1)  OutDataTypeStr=double  SampleTime=Ts
  Input Param. for forwardKinematics and computeJacobians 2 : Constant  Value=zeros(ROBOT_DOF+16,1)  OutDataTypeStr=double  SampleTime=Ts
  Input Param. for forwardKinematics and computeJacobians 3 : Constant  Value=zeros(ROBOT_DOF+6,1)  OutDataTypeStr=double  SampleTime=Ts
  Input Param. for forwardKinematics and computeJacobians 4 : Constant  Value=zeros(ROBOT_DOF+6,1)  OutDataTypeStr=double  SampleTime=Ts
  S-Function : S-Function  FunctionName=robotState  Parameters=val,robotname,localname,linkname  EnableBusSupport=off  mask{val=3, robotname=robotName, localname=localName, linkname='na'}
      mask prompts: val "Value"; robotname "Robot Name (icub - icubSim)"; localname "Module Name"; linkname "Link Name"
  Terminator1 : Terminator
  Terminator2 : Terminator
  Terminator3 : Terminator
  dqrad{,1..5} (6 alike) : Terminator
  massMatrix : Terminator
  massMatrix1 : Terminator
  qrad : Terminator
  Jacobian : Outport
  wires:
  Input Param. for forwardKinematics and computeJacobians 1/1 -> S-Function/2
  S-Function/2 -> dqrad/1
  S-Function/1 -> qrad/1
  S-Function/3 -> Terminator1/1
  "Input Param. for forwardKinematics and computeJacobians "/1 -> S-Function/1
  S-Function/4 -> Jacobian/1
  S-Function/5 -> massMatrix/1
  S-Function/6 -> Terminator3/1
  S-Function/7 -> dqrad1/1
  S-Function/8 -> massMatrix1/1
  S-Function/9 -> Terminator2/1
  S-Function/10 -> dqrad2/1
  Input Param. for forwardKinematics and computeJacobians 2/1 -> S-Function/3
  Input Param. for forwardKinematics and computeJacobians 3/1 -> S-Function/4
  Input Param. for forwardKinematics and computeJacobians 4/1 -> S-Function/5
  S-Function/11 -> dqrad3/1
  S-Function/12 -> dqrad4/1
  S-Function/13 -> dqrad5/1

== system WBCLibrary/wholeBodyModel/Jacobians/Left Hand Jacobian/Left Hand Jacobian ==
  "Input Param. for forwardKinematics and computeJacobians " : Constant  Value=4  OutDataTypeStr=int8  SampleTime=Ts
  Input Param. for forwardKinematics and computeJacobians 1 : Constant  Value=zeros(ROBOT_DOF,1)  OutDataTypeStr=double  SampleTime=Ts
  Input Param. for forwardKinematics and computeJacobians 2 : Constant  Value=zeros(ROBOT_DOF+16,1)  OutDataTypeStr=double  SampleTime=Ts
  Input Param. for forwardKinematics and computeJacobians 3 : Constant  Value=zeros(ROBOT_DOF+6,1)  OutDataTypeStr=double  SampleTime=Ts
  Input Param. for forwardKinematics and computeJacobians 4 : Constant  Value=zeros(ROBOT_DOF+6,1)  OutDataTypeStr=double  SampleTime=Ts
  S-Function : S-Function  FunctionName=robotState  Parameters=val,robotname,localname,linkname  EnableBusSupport=off  mask{val=3, robotname=robotName, localname=localName, linkname='na'}
      mask prompts: val "Value"; robotname "Robot Name (icub - icubSim)"; localname "Module Name"; linkname "Link Name"
  Terminator{1..4} (4 alike) : Terminator
  dqrad{,1..3} (4 alike) : Terminator
  massMatrix : Terminator
  massMatrix1 : Terminator
  massMatrix2 : Terminator
  qrad : Terminator
  Jacobian : Outport
  wires:
  Input Param. for forwardKinematics and computeJacobians 4/1 -> S-Function/5
  Input Param. for forwardKinematics and computeJacobians 3/1 -> S-Function/4
  Input Param. for forwardKinematics and computeJacobians 2/1 -> S-Function/3
  S-Function/10 -> dqrad2/1
  S-Function/9 -> Terminator2/1
  S-Function/8 -> massMatrix1/1
  S-Function/7 -> dqrad1/1
  S-Function/6 -> Terminator3/1
  S-Function/5 -> massMatrix/1
  S-Function/4 -> Jacobian/1
  "Input Param. for forwardKinematics and computeJacobians "/1 -> S-Function/1
  S-Function/3 -> Terminator1/1
  S-Function/1 -> qrad/1
  S-Function/2 -> dqrad/1
  Input Param. for forwardKinematics and computeJacobians 1/1 -> S-Function/2
  S-Function/13 -> dqrad3/1
  S-Function/12 -> Terminator4/1
  S-Function/11 -> massMatrix2/1

== system WBCLibrary/wholeBodyModel/Jacobians/Link Jacobian/Link Jacobian ==
  "Input Param. for forwardKinematics and computeJacobians " : Constant  OutDataTypeStr=int8  SampleTime=Ts
  Input Param. for forwardKinematics and computeJacobians 1 : Constant  Value=zeros(ROBOT_DOF,1)  OutDataTypeStr=double  SampleTime=Ts
  Input Param. for forwardKinematics and computeJacobians 2 : Constant  Value=zeros(ROBOT_DOF+16,1)  OutDataTypeStr=double  SampleTime=Ts
  Input Param. for forwardKinematics and computeJacobians 3 : Constant  Value=zeros(ROBOT_DOF+6,1)  OutDataTypeStr=double  SampleTime=Ts
  Input Param. for forwardKinematics and computeJacobians 4 : Constant  Value=zeros(ROBOT_DOF+6,1)  OutDataTypeStr=double  SampleTime=Ts
  S-Function : S-Function  FunctionName=robotState  Parameters=val,robotname,localname,LinkName  EnableBusSupport=off  mask{val=18, robotname=robotname, localname=localname, linkname=LinkName}
      mask prompts: val "Value"; robotname "Robot Name (icub - icubSim)"; localname "Module Name"; linkname "Link Name"
  Terminator1 : Terminator
  Terminator2 : Terminator
  Terminator3 : Terminator
  dqrad{,1..5} (6 alike) : Terminator
  massMatrix : Terminator
  massMatrix1 : Terminator
  qrad : Terminator
  Jacobian : Outport
  wires:
  S-Function/13 -> dqrad5/1
  S-Function/12 -> dqrad4/1
  S-Function/11 -> dqrad3/1
  Input Param. for forwardKinematics and computeJacobians 4/1 -> S-Function/5
  Input Param. for forwardKinematics and computeJacobians 3/1 -> S-Function/4
  Input Param. for forwardKinematics and computeJacobians 2/1 -> S-Function/3
  S-Function/10 -> dqrad2/1
  S-Function/9 -> Terminator2/1
  S-Function/8 -> massMatrix1/1
  S-Function/7 -> dqrad1/1
  S-Function/6 -> Terminator3/1
  S-Function/5 -> massMatrix/1
  S-Function/4 -> Jacobian/1
  "Input Param. for forwardKinematics and computeJacobians "/1 -> S-Function/1
  S-Function/3 -> Terminator1/1
  S-Function/1 -> qrad/1
  S-Function/2 -> dqrad/1
  Input Param. for forwardKinematics and computeJacobians 1/1 -> S-Function/2

== system WBCLibrary/wholeBodyModel/Jacobians/Right Foot Jacobian/Right Foot Jacobian ==
  "Input Param. for forwardKinematics and computeJacobians " : Constant  Value=0  OutDataTypeStr=int8  SampleTime=Ts
  Input Param. for forwardKinematics and computeJacobians 1 : Constant  Value=zeros(ROBOT_DOF,1)  OutDataTypeStr=double  SampleTime=Ts
  Input Param. for forwardKinematics and computeJacobians 2 : Constant  Value=zeros(ROBOT_DOF+16,1)  OutDataTypeStr=double  SampleTime=Ts
  Input Param. for forwardKinematics and computeJacobians 3 : Constant  Value=zeros(ROBOT_DOF+6,1)  OutDataTypeStr=double  SampleTime=Ts
  Input Param. for forwardKinematics and computeJacobians 4 : Constant  Value=zeros(ROBOT_DOF+6,1)  OutDataTypeStr=double  SampleTime=Ts
  S-Function : S-Function  FunctionName=robotState  Parameters=val,robotname,localname,linkname  EnableBusSupport=off  mask{val=3, robotname=robotName, localname=localName, linkname='na'}
      mask prompts: val "Value"; robotname "Robot Name (icub - icubSim)"; localname "Module Name"; linkname "Link Name"
  Terminator{1..8} (8 alike) : Terminator
  dqRad : Terminator
  massMatrix : Terminator
  qRad : Terminator
  x : Terminator
  Jacobian : Outport
  wires:
  Input Param. for forwardKinematics and computeJacobians 1/1 -> S-Function/2
  S-Function/4 -> Jacobian/1
  "Input Param. for forwardKinematics and computeJacobians "/1 -> S-Function/1
  S-Function/3 -> x/1
  S-Function/1 -> qRad/1
  S-Function/2 -> dqRad/1
  S-Function/5 -> massMatrix/1
  S-Function/6 -> Terminator4/1
  S-Function/7 -> Terminator5/1
  S-Function/8 -> Terminator1/1
  S-Function/9 -> Terminator2/1
  S-Function/10 -> Terminator3/1
  Input Param. for forwardKinematics and computeJacobians 2/1 -> S-Function/3
  Input Param. for forwardKinematics and computeJacobians 3/1 -> S-Function/4
  Input Param. for forwardKinematics and computeJacobians 4/1 -> S-Function/5
  S-Function/11 -> Terminator6/1
  S-Function/12 -> Terminator7/1
  S-Function/13 -> Terminator8/1

== system WBCLibrary/wholeBodyModel/Jacobians/Right Hand Jacobian/Right Hand Jacobian ==
  "Input Param. for forwardKinematics and computeJacobians " : Constant  Value=3  OutDataTypeStr=int8  SampleTime=Ts
  Input Param. for forwardKinematics and computeJacobians 1 : Constant  Value=zeros(ROBOT_DOF,1)  OutDataTypeStr=double  SampleTime=Ts
  Input Param. for forwardKinematics and computeJacobians 2 : Constant  Value=zeros(ROBOT_DOF+16,1)  OutDataTypeStr=double  SampleTime=Ts
  Input Param. for forwardKinematics and computeJacobians 3 : Constant  Value=zeros(ROBOT_DOF+6,1)  OutDataTypeStr=double  SampleTime=Ts
  Input Param. for forwardKinematics and computeJacobians 4 : Constant  Value=zeros(ROBOT_DOF+6,1)  OutDataTypeStr=double  SampleTime=Ts
  S-Function : S-Function  FunctionName=robotState  Parameters=val,robotname,localname,linkname  EnableBusSupport=off  mask{val=3, robotname=robotName, localname=localName, linkname='na'}
      mask prompts: val "Value"; robotname "Robot Name (icub - icubSim)"; localname "Module Name"; linkname "Link Name"
  Terminator{1..8} (8 alike) : Terminator
  dqRad : Terminator
  massMatrix : Terminator
  qRad : Terminator
  x : Terminator
  Jacobian : Outport
  wires:
  Input Param. for forwardKinematics and computeJacobians 4/1 -> S-Function/5
  Input Param. for forwardKinematics and computeJacobians 3/1 -> S-Function/4
  Input Param. for forwardKinematics and computeJacobians 2/1 -> S-Function/3
  S-Function/10 -> Terminator3/1
  S-Function/9 -> Terminator2/1
  S-Function/8 -> Terminator1/1
  S-Function/7 -> Terminator5/1
  S-Function/6 -> Terminator4/1
  S-Function/5 -> massMatrix/1
  S-Function/2 -> dqRad/1
  S-Function/1 -> qRad/1
  S-Function/3 -> x/1
  "Input Param. for forwardKinematics and computeJacobians "/1 -> S-Function/1
  S-Function/4 -> Jacobian/1
  Input Param. for forwardKinematics and computeJacobians 1/1 -> S-Function/2
  S-Function/11 -> Terminator6/1
  S-Function/12 -> Terminator7/1
  S-Function/13 -> Terminator8/1

== matlab function WBCLibrary/Utilities/holder /MATLAB Function ==
  data: s input; s0 output; t input
function s0 = fcn(s, t)
persistent state
%#codegen


if isempty(state)
    state = s;
    s
end

s0 = state;

== matlab function WBCLibrary/Utilities/baseVelocity/MATLAB Function ==
  data: JcIn input; y output; qD input
function y = fcn(JcIn, qD)
%#codegen
y = -pinv(JcIn(:,1:6))*JcIn(:,7:end)*qD;

== matlab function WBCLibrary/Utilities/DampPinv/Damped Pseudo Inverse ==
  data: mat input; DPinv output; sigma input
function DPinv  = fcn(mat,sigma)
% Economody size svd of mat
[U,S,V] = svd(mat,'econ');
% Damped version of S with sigma
S(S>sigma)=S(S>sigma)./((S(S>sigma)).^2+sigma^2);
% Damped pseudoinverse
DPinv = V*pinv(S)*U';

== matlab function WBCLibrary/Utilities/TruncPinv/Truncated PseudoInverse ==
  data: mat input; TPinv output; tol input
function TPinv  = fcn(mat,tol)
%#codegen
[U,S,V] = svd(mat,'econ');
% Setting to zero value
% Setting to 1/S(i,i) singular values greater than tol
 S(S>tol)=1./S(S>tol);
 TPinv = V*pinv(S)*U';
